simulink model "interface"  (R2018b)
settings: Solver=FixedStepDiscrete  StartTime=0.0  StopTime=10.0  RelTol=1e-3
settings Model: Creator=matlab  LastModifiedBy=matlab

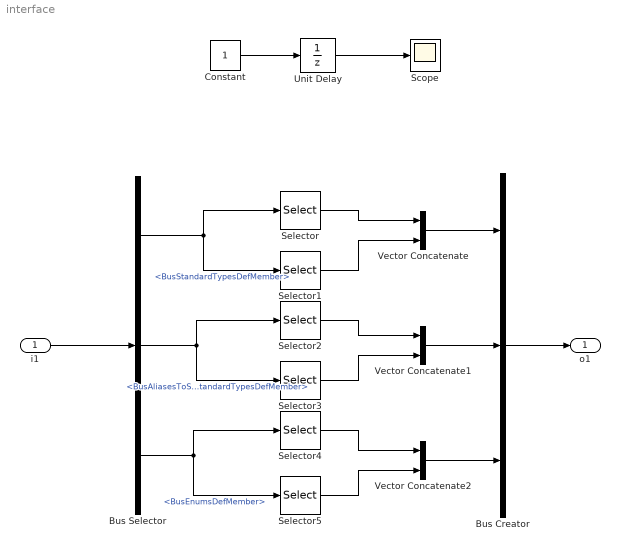
== system interface ==
  i1 : Inport  OutDataTypeStr=Bus: BusDef  BusOutputAsStruct=on
  Bus Creator : BusCreator  Inputs=3  OutDataTypeStr=Bus: BusDef  NonVirtualBus=on
  Bus Selector : BusSelector  OutputSignals=BusStandardTypesDefMember,BusAliasesToStandardTypesDefMember,BusEnumsDefMember
  Constant : Constant
  Scope : Scope
  Selector : Selector  InputPortWidth=2  IndexOptions=Index vector (dialog)  Indices=1  OutputSizes=1
  Selector1 : Selector  InputPortWidth=2  IndexOptions=Index vector (dialog)  Indices=2  OutputSizes=1
  Selector2 : Selector  InputPortWidth=2  IndexOptions=Index vector (dialog)  Indices=1  OutputSizes=1
  Selector3 : Selector  InputPortWidth=2  IndexOptions=Index vector (dialog)  Indices=2  OutputSizes=1
  Selector4 : Selector  InputPortWidth=2  IndexOptions=Index vector (dialog)  Indices=1  OutputSizes=1
  Selector5 : Selector  InputPortWidth=2  IndexOptions=Index vector (dialog)  Indices=2  OutputSizes=1
  Unit Delay : UnitDelay  SampleTime=-1
  Vector Concatenate : Concatenate
  Vector Concatenate1 : Concatenate
  Vector Concatenate2 : Concatenate
  o1 : Outport  OutDataTypeStr=Bus: BusDef
  wires:
  Unit Delay/1 -> Scope/1
  Constant/1 -> Unit Delay/1
  i1/1 -> Bus Selector/1
  Bus Selector/3 -> Selector5/1, Selector4/1  "<BusEnumsDefMember>"
  Bus Selector/2 -> Selector3/1, Selector2/1  "<BusAliasesToStandardTypesDefMember>"
  Bus Selector/1 -> Selector1/1, Selector/1  "<BusStandardTypesDefMember>"
  Selector/1 -> Vector Concatenate/1
  Selector1/1 -> Vector Concatenate/2
  Vector Concatenate/1 -> Bus Creator/1
  Selector2/1 -> Vector Concatenate1/1
  Vector Concatenate1/1 -> Bus Creator/2
  Selector3/1 -> Vector Concatenate1/2
  Selector4/1 -> Vector Concatenate2/1
  Selector5/1 -> Vector Concatenate2/2
  Vector Concatenate2/1 -> Bus Creator/3
  Bus Creator/1 -> o1/1
